simulink model "problem_1"  (R2020b)
settings: Solver=VariableStepAuto  StartTime=0.0  StopTime=10.0  RelTol=1e-3
settings Model: Creator=hp  LastModifiedBy=hp

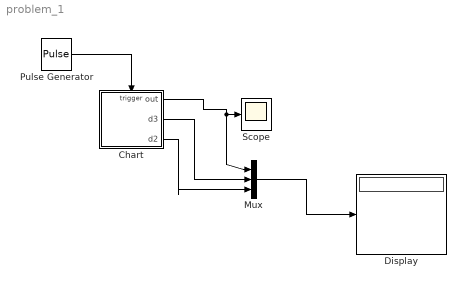
== system problem_1 ==
  Chart : Stateflow chart  TreatAsAtomicUnit=on
  Display : Display
  Mux : Mux  Inputs=3
  Pulse Generator : DiscretePulseGenerator  PulseType=Time based  Period=1  PulseWidth=50
  Scope : Scope
  wires:
  Chart/3(d2) -> Mux/3
  Pulse Generator/1 -> Chart/Trigger
  Mux/1 -> Display/1
  Chart/2(d3) -> Mux/2
  Chart/1(out) -> Mux/1, Scope/1

== stateflow chart problem_1/Chart ==
  state state1 [parallel]
    settings: executionOrder=1
    state one
      en:
      out=1;
    state zero
      en:
      out=0;
    state two
      en:
      out=2;
    state four
      en:
      out=4;
    state three
      en:
      out=3;
    zero -> one : click
    one -> two : click
    (default) -> zero
    four -> zero : click/{state2.event2}
    two -> three : click
    three -> four : click
  state state2 [parallel]
    settings: executionOrder=2
    state one2
      en:
      d2=1;
    state zero2
      en:
      d2=0;
    state two2
      en:
      d2=2;
    state four4
      en:
      d2=4;
    state three3
      en:
      d2=3;
    zero2 -> one2 : event2
    one2 -> two2 : event2
    (default) -> zero2
    state2.four4 -> zero2 : event2/{state3.event3}
    two2 -> state2.three3 : event2
    state2.three3 -> state2.four4 : event2
  state state3 [parallel]
    settings: executionOrder=3
    state one3
      en:
      d3=1;
    state zero3
      en:
      d3=0;
    state two3
      en:
      d3=2;
    state four4
      en:
      d3=4;
    state three3
      en:
      d3=3;
    zero3 -> one3 : event3
    one3 -> two3 : event3
    (default) -> zero3
    state3.four4 -> zero3 : event3
    two3 -> state3.three3 : event3
    state3.three3 -> state3.four4 : event3
  data: out output; d3 output; d2 output
  events: event2 local FUNCTION_CALL_EVENT; event3 local FUNCTION_CALL_EVENT; click input RISING_EDGE_EVENT
